simulink model "pmsm_fpga"  (R2020b)
settings: Solver=FixedStepDiscrete  StartTime=0.0  StopTime=5  FixedStep=1e-5  RelTol=1e-3
PostLoadFcn:
  | try
  | cell = struct2cell(dir(fullfile(speedgoatroot_hdlb, 'hdlsrc', 'pwm', '*.vhd')));
  | addSourceFiles = strjoin(fullfile(cell(2,:),cell(1,:)), ';');
  | hdlset_param('pwm_example_hdlc/DUT PWM and CAP', 'IPCoreAdditionalFiles', addSourceFiles);
  | end
undefined symbols (not defined in the file): J, Tmax, Ts, Tsc
libraries: fl_lib x10, nesl_utility x8, ee_lib x3, simulink x2, quadrature_cpulib x1, pwm_fpgalib x1, quadrature_fpgalib x1, eePmsmFieldOrientedControl x1, pwm_cpulib x1, eeQuadratureDecoder x1, mcbplantlib x1
settings Model: ModifiedByFormat=Speedgoat GmbH  Creator=Speedgoat GmbH  LastModifiedBy=Speedgoat GmbH
settings DataIOCC: LimitDataPoints=on  SaveFormat=Array  ReturnWorkspaceOutputs=off
settings OptimizationCC: BlockReduction=off  ConditionallyExecuteInputs=off  DefaultParameterBehavior=Inlined  LifeSpan=inf
settings DebuggingCC: AlgebraicLoopMsg=error  UnderspecifiedInitializationDetection=Classic  MergeDetectMultiDrivingBlocksExec=none  SolverPrmCheckMsg=warning  InheritedTsInSrcMsg=none  SingleTaskRateTransMsg=error  ParameterPrecisionLossMsg=none  PregeneratedLibrarySubsystemCodeDiagnostic=none  SFUnexpectedBacktrackingDiag=warning  SFNoUnconditionalDefaultTransitionDiag=warning  SFExecutionAtInitializationDiag=none  ArithmeticOperatorsInVariantConditions=warning
settings HardwareCC: ProdBitPerPointer=32  ProdBitPerSizeT=32  ProdBitPerPtrDiffT=32  ProdLargestAtomicFloat=None  ProdIntDivRoundTo=Undefined  ProdEndianess=Unspecified  ProdWordSize=32  ProdHWDeviceType=ASIC/FPGA->ASIC/FPGA  ProdEqTarget=off
settings ModelReferenceCC: PropagateSignalLabelsOutOfModel=off
settings SFSimCC: SimUseLocalCustomCode=off  CustomCodeUndefinedFunction=UseInterfaceOnly
settings RTWCC: RTWUseLocalCustomCode=off
settings CodeAppCC: StateflowObjectComments=on
settings GRTTargetCC: TargetLangStandard=C89/C90 (ANSI)
settings ConfigComp: CovMetricSettings=dw  CovSaveCumulativeToWorkspaceVar=on  CovSaveSingleToWorkspaceVar=on  CovExternalEMLEnable=off

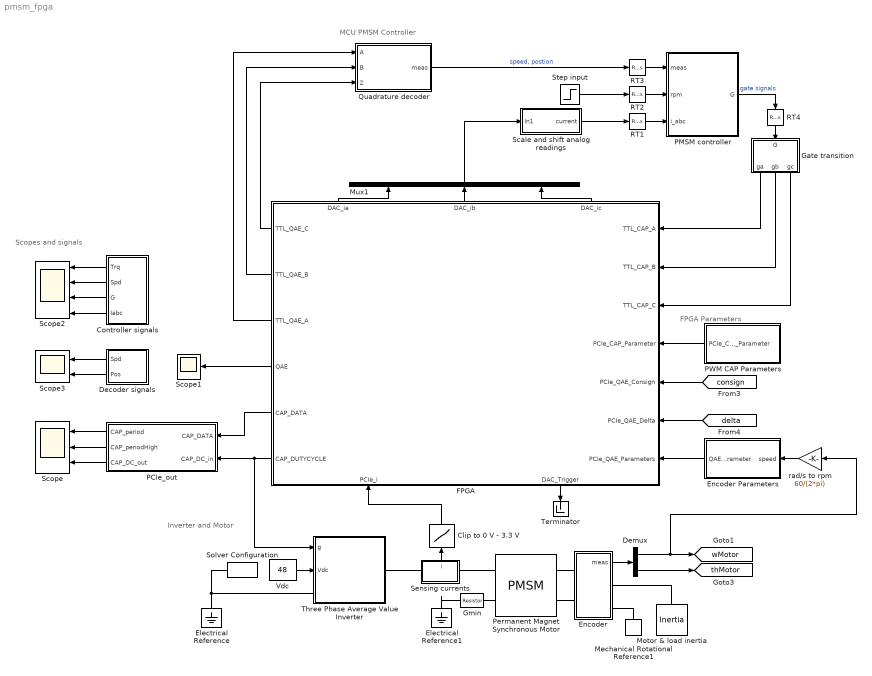
== system pmsm_fpga ==
  note: Scopes and signals
  note: Inverter and Motor
  note: FPGA Parameters
  note: MCU PMSM Controller
  Clip to 0 V - 3.3 V : Lookup_n-D  NumberOfTableDimensions=1  BreakpointsForDimension1=[0, 3.3/10*(2^15-1)]  Table=[0, 3.3/10*(2^15-1)]  ExtrapMethod=Clip  InternalRulePriority=Speed  RndMeth=Simplest  InputSameDT=on
  Controller signals : Subsystem
  Decoder signals : Subsystem
  Demux : Demux  Outputs=2
  Electrical Reference : fl_lib/Electrical/Electrical Elements/Electrical Reference
      settings: SourceProductName=Foundation Library
  Electrical Reference1 : fl_lib/Electrical/Electrical Elements/Electrical Reference
      settings: SourceProductName=Foundation Library
  Encoder : Subsystem
  Encoder Parameters : Subsystem
  FPGA : Subsystem
      settings: PortSchema="{\"entries\":[{\"content\":{\"sides\":[{\"content\":{\"connectorIds\":[\"Out5\",\"Out6\",\"Out7\",\"Out8\",\"Out9\",\"Out10\"]},\"type\":\"ConnectorPlacement.EquallySpacedRectSide\",\"uuid\":\"34ddc533-e92e-4f84-ab54-56ee31c34ed5\"},{\"content\":{\"connectorIds\":[\"In2\",\"In3\",\"In4\",\"In5\",\"In6\",\"In7\",\"In8\"],\"side\":\"RIGHT\"},\"type\":\"ConnectorPlacement.EquallySpacedRectSide\",\"uuid\":\"fc43732f-8b85-47c9-af73-b87840a05fb5\"},{\"content\":{\"connectorIds\":[\"Out2\",\"Out3\",\"Out4\"],\"side\":\"TOP\"},\"type\":\"ConnectorPlacement.EquallySpacedRectSide\",\"uuid\":\"bf663b9c-33b6-4726-afdb-56df835214b8\"},{\"content\":{\"connectorIds\":[\"In1\",\"Out1\"],\"side\":\"BOTTOM\"},\"type\":\"ConnectorPlacement.EquallySpacedRectSide\",\"uuid\":\"04fbffa8-14ef-4425-a219-a420a37a7cbf\"},{\"content\":{\"connectorIds\":[],\"side\":\"HIDDEN\"},\"type\":\"ConnectorPlacement.EquallySpacedRectSide\",\"uuid\":\"ed9b2637-afe7-435a-b994-99eac90c9c32\"}]},\"type\":\"ConnectorPlacement.EquallySpacedConnector\",\"uuid\":\"b4b9272a-3f4d-4e79-a573-4a3ad4933ba9\"}],\"packageUris\":[\"http://schema.mathworks.com/mf0/Connector/R2020b\"],\"version\":\"1.0\"}"
  Gate transition : Subsystem
  Gmin : fl_lib/Electrical/Electrical Elements/Resistor  R=1e6 Ohm  i_specify=off  i_priority=High  i=0 A  i_nominal_specify=off  i_nominal_unit=A  i_nominal_value=1  v_specify=off  v_priority=High  v=0 V  v_nominal_specify=off  v_nominal_unit=V  v_nominal_value=1
      settings: SourceProductName=Foundation Library
  Mechanical Rotational Reference1 : fl_lib/Mechanical/Rotational Elements/Mechanical Rotational Reference
      settings: SourceProductName=Foundation Library
  Motor & load inertia : fl_lib/Mechanical/Rotational Elements/Inertia  inertia=J kg*m^2  num_ports=foundation.enum.numPorts2.one  w_specify=on  w_priority=High  w=0 rpm  w_nominal_specify=off  w_nominal_unit=rad/s  w_nominal_value=1  t_specify=off  t_priority=High  t=0 N*m  t_nominal_specify=off  t_nominal_unit=N*m  t_nominal_value=1
      settings: SourceProductName=Foundation Library
  Mux1 : Mux  Inputs=3
  PCIe_out : Subsystem
  PMSM controller : Subsystem
  PWM CAP Parameters : Subsystem
  Permanent Magnet Synchronous Motor : ee_lib/Electromechanical/Permanent Magnet/PMSM  winding_type=ee.enum.statorconnection.wye  machine_param=ee.enum.pmsm.parameterization.constant  nPolePairs=N  pmflux_param=ee.enum.pmflux.fluxlinkage  pm_flux_linkage=PM Wb  torque_constant=0.18 N*m/A  back_emf_constant=0.18 V/(rad/s)  stator_param=ee.enum.statorparam.LdLqL0  Ld=Ld H  Lq=Lq H  idVec=[-200, 0, 200] A  iqVec=[-200, 0, 200] A  LdMatrix=0.0002 * ones(3, 3) H  LqMatrix=0.0002 * ones(3, 3) H  PmMatrix=0.1 * ones(3, 3) Wb  ktMatrix=0.18 * ones(3, 3) N*m/A  keMatrix=0.18 * ones(3, 3) V/(rad/s)  L0=L0 H  Ls=0.0002 H  Lm=0.00002 H  Ms=0.00002 H  Rs=Rs Ohm  zero_sequence=ee.enum.park.zerosequence.exclude  J=0 kg*m^2  lam=0 N*m/(rad/s)  axes_param=ee.enum.rotorangle.qaxis  i_d_specify=off  i_d_priority=None  i_d=0 A  i_d_nominal_specify=off  i_d_nominal_unit=A  i_d_nominal_value=1  i_q_specify=off  i_q_priority=None  i_q=0 A  i_q_nominal_specify=off  i_q_nominal_unit=A  i_q_nominal_value=1  torque_specify=off  torque_priority=None  torque=0 N*m  torque_nominal_specify=off  torque_nominal_unit=N*m  torque_nominal_value=1  angular_velocity_specify=on  angular_velocity_priority=None  angular_velocity=0 rpm  angular_velocity_nominal_specify=off  angular_velocity_nominal_unit=rpm  angular_velocity_nominal_value=1  angular_position_specify=on  angular_position_priority=High  angular_position=0 rad  angular_position_nominal_specify=off  angular_position_nominal_unit=deg  angular_position_nominal_value=1  loss_param=ee.enum.ironloss.none  losses_oc=[0, 0, 0] W  losses_sc=[0, 0, 0] W  f_losses=60 Hz  Isc_losses=95 A  Tmeas=298.15 K  alpha=3.93e-3 1/K  alpha_flux=-0.001 1/K  stator_thermal_mass=100 J/K  rotor_thermal_mass=200 J/K  Rm_percent_rotor=90  Rd_percent_rotor=30  temperatureA_specify=off  temperatureA_priority=High  temperatureA=25 degC  temperatureA_nominal_specify=off  temperatureA_nominal_unit=degC  temperatureA_nominal_value=1  temperatureB_specify=off  temperatureB_priority=High  temperatureB=25 degC  temperatureB_nominal_specify=off  temperatureB_nominal_unit=degC  temperatureB_nominal_value=1  temperatureC_specify=off  temperatureC_priority=High  temperatureC=25 degC  temperatureC_nominal_specify=off  temperatureC_nominal_unit=degC  temperatureC_nominal_value=1  temperatureR_specify=off  temperatureR_priority=High  temperatureR=25 degC  temperatureR_nominal_specify=off  temperatureR_nominal_unit=degC  temperatureR_nominal_value=1
      settings: SourceProductName=Electrical  InternalSimscapePortConfiguration="{\"Bottom\":[],\"Left\":[{\"id\":\"N\",\"label\":\"~\",\"type\":\"foundation.electrical.three_phase\"},{\"id\":\"n\",\"label\":\"n\",\"type\":\"foundation.electrical.electrical\"}],\"Right\":[{\"id\":\"R\",\"label\":\"R\",\"type\":\"foundation.mechanical.rotational.rotational\"},{\"id\":\"C\",\"label\":\"C\",\"type\":\"foundation.mechanical.rotational.rotational\"}],\"Top\":[]}"
  Quadrature decoder : Subsystem
  RT{1..4} (4 alike) : RateTransition  OutPortSampleTime=Tsc
  Scale and shift analog readings : Subsystem
  Scope : Scope  NumInputPorts=3
  Scope1 : Scope
  Scope2 : Scope  NumInputPorts=4
  Scope3 : Scope  NumInputPorts=2
  Sensing currents : Subsystem
      settings: PortSchema="{\"entries\":[{\"content\":{\"sides\":[{\"content\":{\"connectorIds\":[\"LConn1\"]},\"type\":\"ConnectorPlacement.EquallySpacedRectSide\",\"uuid\":\"5944ef88-f0e5-49d7-9ad6-739ca14af38a\"},{\"content\":{\"connectorIds\":[\"RConn1\"],\"side\":\"RIGHT\"},\"type\":\"ConnectorPlacement.EquallySpacedRectSide\",\"uuid\":\"52c09ccb-1303-4088-b38f-68b8aea00489\"},{\"content\":{\"connectorIds\":[\"Out1\"],\"side\":\"TOP\"},\"type\":\"ConnectorPlacement.EquallySpacedRectSide\",\"uuid\":\"f2e54c46-4573-400c-9f21-48a88d224d47\"},{\"content\":{\"connectorIds\":[],\"side\":\"HIDDEN\"},\"type\":\"ConnectorPlacement.EquallySpacedRectSide\",\"uuid\":\"a55d9811-d0ed-49ba-b1a1-43558df722e5\"}]},\"type\":\"ConnectorPlacement.EquallySpacedConnector\",\"uuid\":\"6a30da7c-a08b-4558-b141-c480e5507c55\"}],\"packageUris\":[\"http://schema.mathworks.com/mf0/Connector/R2020b\"],\"version\":\"1.0\"}"
      mask Display: disp('i')
  Solver Configuration : nesl_utility/Solver Configuration  PhysicalDomain=network_engine_domain  SubClassName=solver  LeftPortType=input  RightPortType=generic  Tones=[]  Harmonics=[]  SimulateNoise=off  Profile=off  UseLocalSampling=off  EnableSwitchedLinearOptims=on  FrequencyDomain=off  UseCCode=off  RelTol=0.001  AbsTol=1e-06  MinStep=1e-09  ToWorkspace=off  RevertToSquareIcSolve=off  NumHomotopyIterations=100  PhasorMode=off  PhasorModeNumHarmonics=1  DoDC=off  ResidualTolerance=1e-9  UseLocalSolver=on  LocalSolverChoice=NE_BACKWARD_EULER_ADVANCER  LocalSolverSampleTime=Ts  DoFixedCost=on  MaxNonlinIter=4  MaxModeIter=2  ComputeImpulses=off  ImpulseIterations=2  LinearAlgebra=auto  EquationFormulation=NE_TIME_EF  DelaysMemoryBudget=1024  AutomaticFiltering=on  FilteringTimeConstant=0.001  PartitionStorageMethod=AS_NEEDED  PartitionMemoryBudget=1024  PartitionMethod=FAST
      settings: SourceProductName=Utilities
  Step input : Step  Time=0.1  After=500  SampleTime=Ts
  Terminator : Terminator
  Three Phase Average Value Inverter : Subsystem
  Vdc : Constant  Value=48  SampleTime=Tsc
  rad/s to rpm : Gain  Gain=60/(2*pi)
  tag scope: thMotor=global, wMotor=global
  wires:
  PCIe_out/3(CAP_DC_out) -> Scope/3
  PCIe_out/2(CAP_periodHigh) -> Scope/2
  PCIe_out/1(CAP_period) -> Scope/1
  Encoder Parameters/1(QAE_parameter) -> FPGA/8(PCIe_QAE_Parameters)
  PWM CAP Parameters/1(PCIe_CAP_Parameter) -> FPGA/5(PCIe_CAP_Parameter)
  FPGA/10(CAP_DUTYCYCLE) -> Three Phase Average Value Inverter/1(g), PCIe_out/2(CAP_DC_in)
  FPGA/9(CAP_DATA) -> PCIe_out/1(CAP_DATA)
  Encoder/1(meas) -> Demux/1
  Vdc/1 -> Three Phase Average Value Inverter/2(Vdc)
  Demux/1 -> rad/s to rpm/1, [wMotor]
  Demux/2 -> [thMotor]
  rad/s to rpm/1 -> Encoder Parameters/1(speed)
  FPGA/8(QAE) -> Scope1/1
  RT3/1 -> PMSM controller/1(meas)
  RT2/1 -> PMSM controller/2(rpm)
  RT1/1 -> PMSM controller/3(i_abc)
  Step input/1 -> RT2/1
  FPGA/3(DAC_ib) -> Mux1/2
  FPGA/2(DAC_ia) -> Mux1/1
  FPGA/4(DAC_ic) -> Mux1/3
  FPGA/1(DAC_Trigger) -> Terminator/1
  FPGA/5(TTL_QAE_C) -> Quadrature decoder/3(Z)
  FPGA/6(TTL_QAE_B) -> Quadrature decoder/2(B)
  FPGA/7(TTL_QAE_A) -> Quadrature decoder/1(A)
  Quadrature decoder/1(meas) -> RT3/1  "speed, postion"
  Controller signals/1(Trq) -> Scope2/1
  Controller signals/2(Spd) -> Scope2/2
  Controller signals/4(Iabc) -> Scope2/4
  Controller signals/3(G) -> Scope2/3
  Decoder signals/1(Spd) -> Scope3/1
  Decoder signals/2(Pos) -> Scope3/2
  [delta] -> FPGA/7(PCIe_QAE_Delta)
  [consign] -> FPGA/6(PCIe_QAE_Consign)
  PMSM controller/1(G) -> RT4/1  "gate signals"
  Gate transition/1(ga) -> FPGA/2(TTL_CAP_A)
  Gate transition/2(gb) -> FPGA/3(TTL_CAP_B)
  Gate transition/3(gc) -> FPGA/4(TTL_CAP_C)
  Sensing currents/1(i) -> Clip to 0 V - 3.3 V/1
  Clip to 0 V - 3.3 V/1 -> FPGA/1(PCIe_i)
  Mux1/1 -> Scale and shift analog readings/1(In1)
  Scale and shift analog readings/1(current) -> RT1/1
  RT4/1 -> Gate transition/1(G)
  connections:
  Solver Configuration/RConn1 -- Electrical Reference/LConn1 -- Three Phase Average Value Inverter/LConn1
  Electrical Reference1/LConn1 -- Gmin/LConn1
  Encoder/RConn1 -- Motor & load inertia/LConn1
  Permanent Magnet Synchronous Motor/RConn1 -- Encoder/LConn1
  Three Phase Average Value Inverter/RConn1 -- Sensing currents/LConn1
  Permanent Magnet Synchronous Motor/RConn2 -- Encoder/LConn2
  Mechanical Rotational Reference1/LConn1 -- Encoder/RConn2
  Permanent Magnet Synchronous Motor/LConn1 -- Sensing currents/RConn1
  Gmin/RConn1 -- Permanent Magnet Synchronous Motor/LConn2

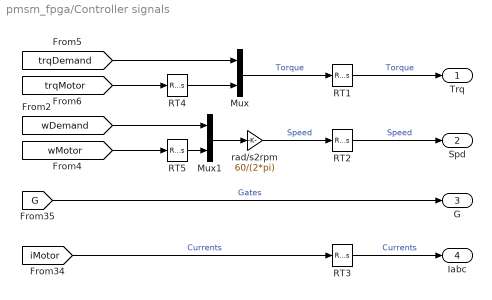
== system pmsm_fpga/Controller signals ==
  Mux : Mux  Inputs=2
  Mux1 : Mux  Inputs=2
  RT1 : RateTransition  OutPortSampleTime=Ts
  RT2 : RateTransition  OutPortSampleTime=Ts
  RT3 : RateTransition  OutPortSampleTime=Ts
  RT4 : RateTransition  OutPortSampleTime=Tsc
  RT5 : RateTransition  OutPortSampleTime=Tsc
  rad/s2rpm : Gain  Gain=60/(2*pi)
  Trq : Outport  VectorParamsAs1DForOutWhenUnconnected=off
  Spd : Outport  Port=2  VectorParamsAs1DForOutWhenUnconnected=off
  G : Outport  Port=3  VectorParamsAs1DForOutWhenUnconnected=off
  Iabc : Outport  Port=4  VectorParamsAs1DForOutWhenUnconnected=off
  wires:
  [trqDemand] -> Mux/1
  [G] -> G/1  "Gates"
  Mux1/1 -> rad/s2rpm/1
  Mux/1 -> RT1/1  "Torque"
  [iMotor] -> RT3/1  "Currents"
  [wDemand] -> Mux1/1
  rad/s2rpm/1 -> RT2/1  "Speed"
  [trqMotor] -> RT4/1
  [wMotor] -> RT5/1
  RT1/1 -> Trq/1  "Torque"
  RT2/1 -> Spd/1  "Speed"
  RT3/1 -> Iabc/1  "Currents"
  RT4/1 -> Mux/2
  RT5/1 -> Mux1/2

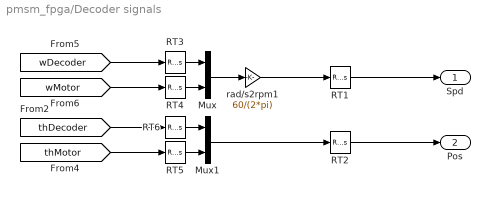
== system pmsm_fpga/Decoder signals ==
  Mux : Mux  Inputs=2
  Mux1 : Mux  Inputs=2
  RT1 : RateTransition  OutPortSampleTime=Ts
  RT2 : RateTransition  OutPortSampleTime=Ts
  RT{3..6} (4 alike) : RateTransition  OutPortSampleTime=Tsc
  rad/s2rpm1 : Gain  Gain=60/(2*pi)
  Spd : Outport  VectorParamsAs1DForOutWhenUnconnected=off
  Pos : Outport  Port=2  VectorParamsAs1DForOutWhenUnconnected=off
  wires:
  [wDecoder] -> RT3/1
  Mux/1 -> rad/s2rpm1/1
  [thDecoder] -> RT6/1
  Mux1/1 -> RT2/1
  [wMotor] -> RT4/1
  [thMotor] -> RT5/1
  RT1/1 -> Spd/1
  RT2/1 -> Pos/1
  RT4/1 -> Mux/2
  RT5/1 -> Mux1/2
  rad/s2rpm1/1 -> RT1/1
  RT3/1 -> Mux/1
  RT6/1 -> Mux1/1

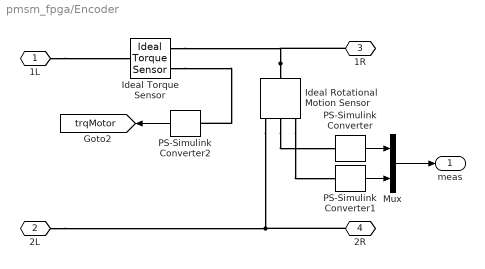
== system pmsm_fpga/Encoder ==
  Ideal Rotational Motion Sensor : fl_lib/Mechanical/Mechanical Sensors/Ideal Rotational Motion Sensor  wrap_angle=simscape.enum.onoff.off  offset=0 deg
      settings: SourceProductName=Foundation Library
  Ideal Torque Sensor : fl_lib/Mechanical/Mechanical Sensors/Ideal Torque Sensor
      settings: SourceProductName=Foundation Library
  Mux : Mux  Inputs=2
  PS-Simulink Converter : nesl_utility/PS-Simulink Converter  PhysicalDomain=network_engine_domain  SubClassName=ps_output  LeftPortType=input  RightPortType=output  PseudoPeriodic=off  Frequencies=[]  Unit=rad/s  AffineConversion=off
      settings: SourceProductName=Utilities
  PS-Simulink Converter1 : nesl_utility/PS-Simulink Converter  PhysicalDomain=network_engine_domain  SubClassName=ps_output  LeftPortType=input  RightPortType=output  PseudoPeriodic=off  Frequencies=[]  Unit=rad  AffineConversion=off
      settings: SourceProductName=Utilities
  PS-Simulink Converter2 : nesl_utility/PS-Simulink Converter  PhysicalDomain=network_engine_domain  SubClassName=ps_output  LeftPortType=input  RightPortType=output  PseudoPeriodic=off  Frequencies=[]  Unit=N*m  AffineConversion=off
      settings: SourceProductName=Utilities
  1L : PMIOPort  Side=Left
  2L : PMIOPort  Port=2  Side=Left
  1R : PMIOPort  Port=3  Side=Right
  2R : PMIOPort  Port=4  Side=Right
  meas : Outport  VectorParamsAs1DForOutWhenUnconnected=off
  tag scope: trqMotor=global
  wires:
  PS-Simulink Converter2/1 -> [trqMotor]
  Mux/1 -> meas/1
  PS-Simulink Converter1/1 -> Mux/2
  PS-Simulink Converter/1 -> Mux/1
  connections:
  Ideal Torque Sensor/RConn2 -- PS-Simulink Converter2/LConn1
  1L/RConn1 -- Ideal Torque Sensor/LConn1
  2R/RConn1 -- 2L/RConn1 -- Ideal Rotational Motion Sensor/RConn1
  Ideal Rotational Motion Sensor/LConn1 -- 1R/RConn1 -- Ideal Torque Sensor/RConn1
  Ideal Rotational Motion Sensor/RConn2 -- PS-Simulink Converter/LConn1
  Ideal Rotational Motion Sensor/RConn3 -- PS-Simulink Converter1/LConn1

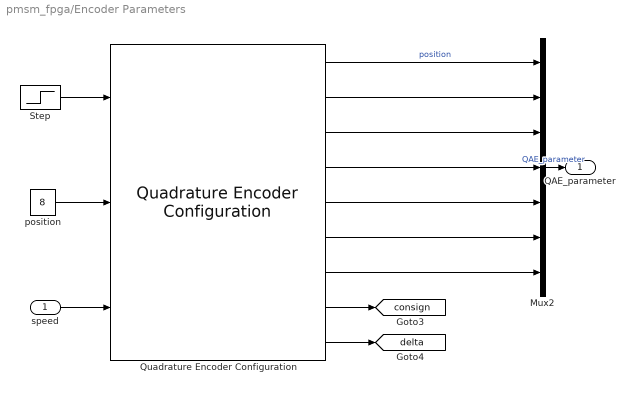
== system pmsm_fpga/Encoder Parameters ==
  speed : Inport
  Mux2 : Mux  Inputs=7
  Quadrature Encoder Configuration : quadrature_cpulib/Quadrature Encoder Configuration  fpgaFreq=100e6  n_channels=1  numSeg=[32]  phaseAngle=90  initPos=[0]  freeWheel=on
      settings: SourceProductName=Simulink Real-Time: Speedgoat HDL Blockset
  Step : Step  Time=0.002
  position : Constant  Value=8  SampleTime=-1
  QAE_parameter : Outport
  tag scope: consign=global, delta=global
  wires:
  speed/1 -> Quadrature Encoder Configuration/3
  Quadrature Encoder Configuration/8 -> [consign]
  Step/1 -> Quadrature Encoder Configuration/1
  Quadrature Encoder Configuration/7 -> Mux2/7
  Quadrature Encoder Configuration/4 -> Mux2/4
  Quadrature Encoder Configuration/2 -> Mux2/2
  position/1 -> Quadrature Encoder Configuration/2
  Mux2/1 -> QAE_parameter/1  "QAE_parameter"
  Quadrature Encoder Configuration/6 -> Mux2/6
  Quadrature Encoder Configuration/5 -> Mux2/5
  Quadrature Encoder Configuration/1 -> Mux2/1  "position"
  Quadrature Encoder Configuration/9 -> [delta]
  Quadrature Encoder Configuration/3 -> Mux2/3

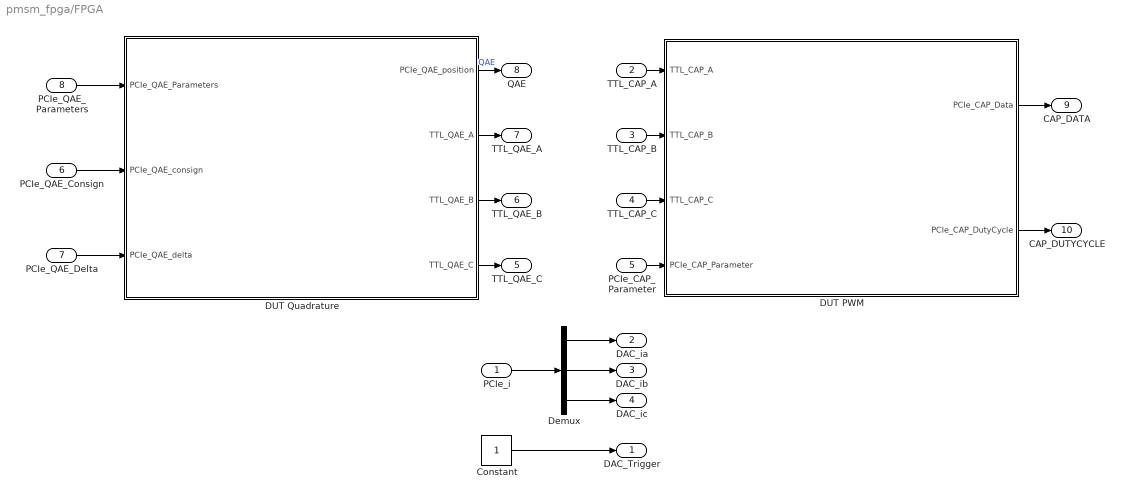
== system pmsm_fpga/FPGA ==
  PCIe_i : Inport  OutDataTypeStr=int16
  TTL_CAP_A : Inport  Port=2
  TTL_CAP_B : Inport  Port=3
  TTL_CAP_C : Inport  Port=4
  PCIe_CAP_Parameter : Inport  Port=5
  PCIe_QAE_Consign : Inport  Port=6
  PCIe_QAE_Delta : Inport  Port=7
  PCIe_QAE_Parameters : Inport  Port=8
  Constant : Constant  OutDataTypeStr=boolean  SampleTime=-1
  DUT PWM : Subsystem
  DUT Quadrature : Subsystem
  Demux : Demux  Outputs=3
  DAC_Trigger : Outport
  DAC_ia : Outport  Port=2
  DAC_ib : Outport  Port=3
  DAC_ic : Outport  Port=4
  TTL_QAE_C : Outport  Port=5
  TTL_QAE_B : Outport  Port=6
  TTL_QAE_A : Outport  Port=7
  QAE : Outport  Port=8
  CAP_DATA : Outport  Port=9
  CAP_DUTYCYCLE : Outport  Port=10
  wires:
  PCIe_QAE_Parameters/1 -> DUT Quadrature/1(PCIe_QAE_Parameters)
  TTL_CAP_B/1 -> DUT PWM/2(TTL_CAP_B)
  PCIe_QAE_Consign/1 -> DUT Quadrature/2(PCIe_QAE_consign)
  PCIe_CAP_Parameter/1 -> DUT PWM/4(PCIe_CAP_Parameter)
  PCIe_QAE_Delta/1 -> DUT Quadrature/3(PCIe_QAE_delta)
  DUT Quadrature/3(TTL_QAE_B) -> TTL_QAE_B/1
  DUT PWM/1(PCIe_CAP_Data) -> CAP_DATA/1
  TTL_CAP_C/1 -> DUT PWM/3(TTL_CAP_C)
  DUT Quadrature/4(TTL_QAE_C) -> TTL_QAE_C/1
  DUT Quadrature/1(PCIe_QAE_position) -> QAE/1  "QAE"
  DUT Quadrature/2(TTL_QAE_A) -> TTL_QAE_A/1
  DUT PWM/2(PCIe_CAP_DutyCycle) -> CAP_DUTYCYCLE/1
  TTL_CAP_A/1 -> DUT PWM/1(TTL_CAP_A)
  PCIe_i/1 -> Demux/1
  Demux/1 -> DAC_ia/1
  Demux/2 -> DAC_ib/1
  Demux/3 -> DAC_ic/1
  Constant/1 -> DAC_Trigger/1

== system pmsm_fpga/Gate transition ==
  G : Inport
  Demux1 : Demux  Outputs=6
  Terminator1 : Terminator
  Terminator2 : Terminator
  Terminator3 : Terminator
  ga : Outport
  gb : Outport  Port=2
  gc : Outport  Port=3
  wires:
  Demux1/2 -> Terminator1/1
  Demux1/6 -> Terminator3/1
  G/1 -> Demux1/1
  Demux1/4 -> Terminator2/1
  Demux1/1 -> ga/1
  Demux1/3 -> gb/1
  Demux1/5 -> gc/1

== system pmsm_fpga/PCIe_out ==
  CAP_DATA : Inport
  CAP_DC_in : Inport  Port=2
  Bus Creator : BusCreator  Inputs=6
  Bus Selector : BusSelector  OutputSignals=PCIe_CAP_Period,PCIe_CAP_periodHigh
  Demux : Demux  Outputs=6
  CAP_period : Outport
  CAP_periodHigh : Outport  Port=2
  CAP_DC_out : Outport  Port=3
  wires:
  CAP_DC_in/1 -> CAP_DC_out/1  "CAP_DutyCycle"
  Bus Selector/2 -> CAP_periodHigh/1  "<PCIe_CAP_periodHigh>"
  Bus Selector/1 -> CAP_period/1  "<PCIe_CAP_Period>"
  Demux/6 -> Bus Creator/6  "PCIe_CAP_Data_Valid"
  Demux/3 -> Bus Creator/3  "PCIe_CAP_periodLow"
  Demux/2 -> Bus Creator/2  "PCIe_CAP_periodHigh"
  Demux/4 -> Bus Creator/4  "PCIe_CAP_TOn"
  Bus Creator/1 -> Bus Selector/1
  Demux/1 -> Bus Creator/1  "PCIe_CAP_Period"
  Demux/5 -> Bus Creator/5  "PCIe_CAP_TOff"
  CAP_DATA/1 -> Demux/1

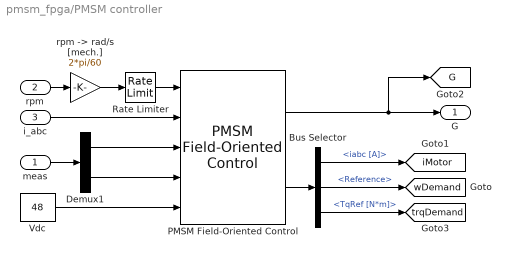
== system pmsm_fpga/PMSM controller ==
  meas : Inport
  rpm : Inport  Port=2
  i_abc : Inport  Port=3
  Bus Selector : BusSelector  OutputSignals=iabc [A],Reference,TqRef [N*m]
  Demux1 : Demux  Outputs=2
  PMSM Field-Oriented Control : eePmsmFieldOrientedControl/PMSM Field-Oriented Control  winding_type=Wye-wound  CtrlMode=Velocity control  Vnom=48  Pmax=Pmax  Tmax=Tmax*1.5  p=N  Vdc_on=10  Ts=Ts  Tsc=Tsc  CtrlType=PI control  Kp_w=60  Ki_w=300*2  Kv_w=1  Kaw_w=1000  RefType=Zero d-axis control  rpmVec=[0, 3000]  TqVec=[-100, 0, 100]  VdcVec=[300, 350]  PWMMode=SPWM: sinusoidal PWM  ModFactor=1  idMatrix=zeros(2,3,2)  iqMatrix=zeros(2,3,2)  psim=PM  Ld=0.00024  Lq=0.00029  Rs=0.01  AxisAlignment=Q-axis  Kp_id=0.1  Ki_id=10  Kaw_id=1000  Kp_iq=0.1  Ki_iq=10  Kaw_iq=1000  AxisPrio=Q-axis  ActZC=off  ActFF=on  ParamTypeFF=Constant parameters  LdFF=Ld  LqFF=Lq  psimFF=PM  idVect=[-200, 0, 200]  iqVect=[-200, 0, 200]  LdMatrix=0.0002 * ones(3, 3)  LqMatrix=0.0002 * ones(3, 3)  psimMatrix=0.04 * ones(3, 3)  CPWMMode=SPWM: sinusoidal PWM  fsw=fsw
      settings: SourceProductBaseCode=PS
  Rate Limiter : RateLimiter  RisingSlewLimit=Tmax/J  FallingSlewLimit=-Tmax/J  SampleTimeMode=inherited
  Vdc : Constant  Value=48  SampleTime=Tsc
  "rpm -> rad/s [mech.]" : Gain  Gain=2*pi/60
  G : Outport  VectorParamsAs1DForOutWhenUnconnected=off
  tag scope: G=global, iMotor=global, trqDemand=global, wDemand=global
  wires:
  PMSM Field-Oriented Control/1 -> G/1, [G]
  Vdc/1 -> PMSM Field-Oriented Control/5
  PMSM Field-Oriented Control/2 -> Bus Selector/1
  i_abc/1 -> PMSM Field-Oriented Control/2
  meas/1 -> Demux1/1
  Demux1/1 -> PMSM Field-Oriented Control/3
  Demux1/2 -> PMSM Field-Oriented Control/4
  Bus Selector/1 -> [iMotor]  "<iabc [A]>"
  Bus Selector/2 -> [wDemand]  "<Reference>"
  Bus Selector/3 -> [trqDemand]  "<TqRef [N*m]>"
  rpm/1 -> "rpm -> rad/s [mech.]"/1
  Rate Limiter/1 -> PMSM Field-Oriented Control/1
  "rpm -> rad/s [mech.]"/1 -> Rate Limiter/1

== system pmsm_fpga/PWM CAP Parameters ==
  Data Type Conversion4 : DataTypeConversion  OutDataTypeStr=uint32
  Data Type Conversion5 : DataTypeConversion  OutDataTypeStr=uint32
  Data Type Conversion6 : DataTypeConversion  OutDataTypeStr=uint32
  Mux1 : Mux  Inputs=3
  PWM Capture Configuration : pwm_cpulib/PWM Capture Configuration  FPGA_freq=100e6  n_channels=1  captureMode=High transitions triggered  captureTimeout=0  PWM_pattern_en=off
      settings: SourceProductName=Simulink Real-Time: Speedgoat HDL Blockset
  PCIe_CAP_Parameter : Outport
  wires:
  PWM Capture Configuration/2 -> Data Type Conversion5/1
  Data Type Conversion6/1 -> Mux1/3
  Data Type Conversion5/1 -> Mux1/2
  Data Type Conversion4/1 -> Mux1/1
  PWM Capture Configuration/3 -> Data Type Conversion6/1
  Mux1/1 -> PCIe_CAP_Parameter/1
  PWM Capture Configuration/1 -> Data Type Conversion4/1

== system pmsm_fpga/Quadrature decoder ==
  A : Inport
  B : Inport  Port=2
  Z : Inport  Port=3
  Mux : Mux  Inputs=2
  Quadrature Shaft Decoder : eeQuadratureDecoder/Quadrature Shaft Decoder  NPulse=16  Ts=-1
      settings: SourceProductBaseCode=PS
  meas : Outport
  tag scope: thDecoder=global, wDecoder=global
  wires:
  Z/1 -> Quadrature Shaft Decoder/3
  B/1 -> Quadrature Shaft Decoder/2
  Quadrature Shaft Decoder/1 -> Mux/1, [wDecoder]
  Mux/1 -> meas/1
  Quadrature Shaft Decoder/2 -> Mux/2, [thDecoder]
  A/1 -> Quadrature Shaft Decoder/1

== system pmsm_fpga/Scale and shift analog readings ==
  In1 : Inport
  Data Type Conversion : DataTypeConversion  OutDataTypeStr=double
  Scale to max range : Gain  Gain=20/3.3
  Shift to allow negative current : Bias  Bias=-2^15
  current : Outport
  wires:
  Scale to max range/1 -> Shift to allow negative current/1
  Data Type Conversion/1 -> Scale to max range/1
  In1/1 -> Data Type Conversion/1
  Shift to allow negative current/1 -> current/1  "current"

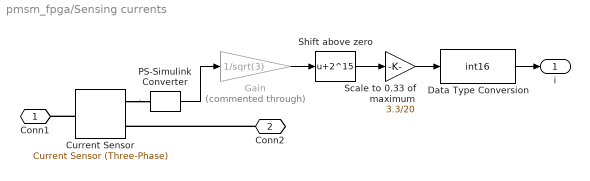
== system pmsm_fpga/Sensing currents ==
  Current Sensor : ee_lib/Sensors & Transducers/Current Sensor (Three-Phase)
      settings: SourceProductName=Electrical
  Data Type Conversion : DataTypeConversion  OutDataTypeStr=int16
  Gain : Gain  Commented=through  Gain=1/sqrt(3)
  PS-Simulink Converter : nesl_utility/PS-Simulink Converter  PhysicalDomain=network_engine_domain  SubClassName=ps_output  LeftPortType=input  RightPortType=output  PseudoPeriodic=off  Frequencies=[]  Unit=A  AffineConversion=off
      settings: SourceProductName=Utilities
  Scale to 0.33 of maximum : Gain  Gain=3.3/20
  Shift above zero : Bias  Bias=2^15
  Conn1 : PMIOPort  Side=Left
  Conn2 : PMIOPort  Port=2  Side=Right
  i : Outport
  wires:
  PS-Simulink Converter/1 -> Gain/1
  Scale to 0.33 of maximum/1 -> Data Type Conversion/1
  Data Type Conversion/1 -> i/1
  Gain/1 -> Shift above zero/1
  Shift above zero/1 -> Scale to 0.33 of maximum/1
  connections:
  Current Sensor/RConn1 -- PS-Simulink Converter/LConn1
  Conn2/RConn1 -- Current Sensor/RConn2
  Current Sensor/LConn1 -- Conn1/RConn1

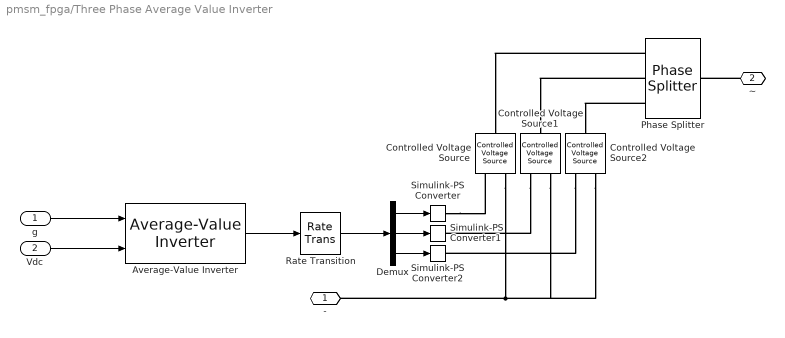
== system pmsm_fpga/Three Phase Average Value Inverter ==
  g : Inport
  Vdc : Inport  Port=2
  Average-Value Inverter : mcbplantlib/Average-Value Inverter
  Controlled Voltage Source : fl_lib/Electrical/Electrical Sources/Controlled Voltage Source
  Controlled Voltage Source1 : fl_lib/Electrical/Electrical Sources/Controlled Voltage Source
  Controlled Voltage Source2 : fl_lib/Electrical/Electrical Sources/Controlled Voltage Source
  Demux : Demux  Outputs=3
  Phase Splitter : ee_lib/Connectors & References/Phase Splitter
      settings: SourceProductBaseCode=PS
  Rate Transition : RateTransition
  Simulink-PS Converter : nesl_utility/Simulink-PS Converter  PhysicalDomain=network_engine_domain  SubClassName=ps_input  LeftPortType=input  RightPortType=output  PseudoPeriodic=off  Frequencies=[]  NoiseDistribution=none  NoiseParameters=[]  Unit=1  AffineConversion=off  FilteringAndDerivatives=provide  SimscapeFilterOrder=1  InputFilterTimeConstant=0.001  UdotUserProvided=0
  Simulink-PS Converter1 : nesl_utility/Simulink-PS Converter  PhysicalDomain=network_engine_domain  SubClassName=ps_input  LeftPortType=input  RightPortType=output  PseudoPeriodic=off  Frequencies=[]  NoiseDistribution=none  NoiseParameters=[]  Unit=1  AffineConversion=off  FilteringAndDerivatives=provide  SimscapeFilterOrder=1  InputFilterTimeConstant=0.001  UdotUserProvided=0
  Simulink-PS Converter2 : nesl_utility/Simulink-PS Converter  PhysicalDomain=network_engine_domain  SubClassName=ps_input  LeftPortType=input  RightPortType=output  PseudoPeriodic=off  Frequencies=[]  NoiseDistribution=none  NoiseParameters=[]  Unit=1  AffineConversion=off  FilteringAndDerivatives=provide  SimscapeFilterOrder=1  InputFilterTimeConstant=0.001  UdotUserProvided=0
  - : PMIOPort  Tag=PMCPort  Side=Left
  ~ : PMIOPort  Tag=PMCPort  Port=2  Side=Right
  wires:
  Demux/3 -> Simulink-PS Converter2/1
  Vdc/1 -> Average-Value Inverter/2
  Demux/2 -> Simulink-PS Converter1/1
  Demux/1 -> Simulink-PS Converter/1
  g/1 -> Average-Value Inverter/1
  Rate Transition/1 -> Demux/1
  Average-Value Inverter/1 -> Rate Transition/1
  connections:
  ~/RConn1 -- Phase Splitter/LConn1
  Controlled Voltage Source/RConn2 -- -/RConn1 -- Controlled Voltage Source1/RConn2 -- Controlled Voltage Source2/RConn2
  Simulink-PS Converter/RConn1 -- Controlled Voltage Source/RConn1
  Controlled Voltage Source2/RConn1 -- Simulink-PS Converter2/RConn1
  Phase Splitter/RConn3 -- Controlled Voltage Source2/LConn1
  Phase Splitter/RConn1 -- Controlled Voltage Source/LConn1
  Phase Splitter/RConn2 -- Controlled Voltage Source1/LConn1
  Controlled Voltage Source1/RConn1 -- Simulink-PS Converter1/RConn1

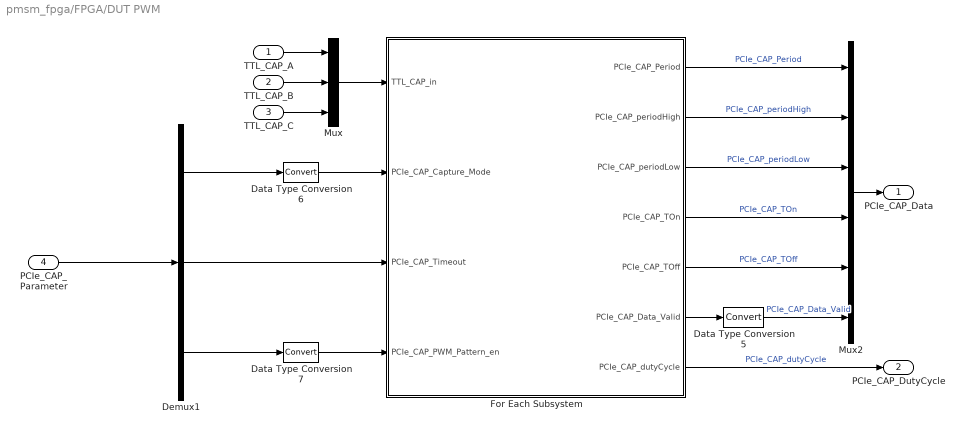
== system pmsm_fpga/FPGA/DUT PWM ==
  TTL_CAP_A : Inport
  TTL_CAP_B : Inport  Port=2
  TTL_CAP_C : Inport  Port=3
  PCIe_CAP_Parameter : Inport  Port=4
  Data Type Conversion5 : DataTypeConversion
  Data Type Conversion6 : DataTypeConversion
  Data Type Conversion7 : DataTypeConversion
  Demux1 : Demux  Outputs=3
  For Each Subsystem : Subsystem  TreatAsAtomicUnit=on
  Mux : Mux  Inputs=3
  Mux2 : Mux  Inputs=6
  PCIe_CAP_Data : Outport  VectorParamsAs1DForOutWhenUnconnected=off
  PCIe_CAP_DutyCycle : Outport  Port=2  VectorParamsAs1DForOutWhenUnconnected=off
  wires:
  Demux1/1 -> Data Type Conversion6/1
  TTL_CAP_A/1 -> Mux/1
  For Each Subsystem/7(PCIe_CAP_dutyCycle) -> PCIe_CAP_DutyCycle/1  "PCIe_CAP_dutyCycle"
  Demux1/2 -> For Each Subsystem/3(PCIe_CAP_Timeout)
  Demux1/3 -> Data Type Conversion7/1
  For Each Subsystem/6(PCIe_CAP_Data_Valid) -> Data Type Conversion5/1
  For Each Subsystem/5(PCIe_CAP_TOff) -> Mux2/5  "PCIe_CAP_TOff"
  For Each Subsystem/4(PCIe_CAP_TOn) -> Mux2/4  "PCIe_CAP_TOn"
  For Each Subsystem/3(PCIe_CAP_periodLow) -> Mux2/3  "PCIe_CAP_periodLow"
  For Each Subsystem/1(PCIe_CAP_Period) -> Mux2/1  "PCIe_CAP_Period"
  For Each Subsystem/2(PCIe_CAP_periodHigh) -> Mux2/2  "PCIe_CAP_periodHigh"
  Mux/1 -> For Each Subsystem/1(TTL_CAP_in)
  TTL_CAP_B/1 -> Mux/2
  Mux2/1 -> PCIe_CAP_Data/1
  Data Type Conversion5/1 -> Mux2/6  "PCIe_CAP_Data_Valid"
  PCIe_CAP_Parameter/1 -> Demux1/1
  Data Type Conversion6/1 -> For Each Subsystem/2(PCIe_CAP_Capture_Mode)
  Data Type Conversion7/1 -> For Each Subsystem/4(PCIe_CAP_PWM_Pattern_en)
  TTL_CAP_C/1 -> Mux/3

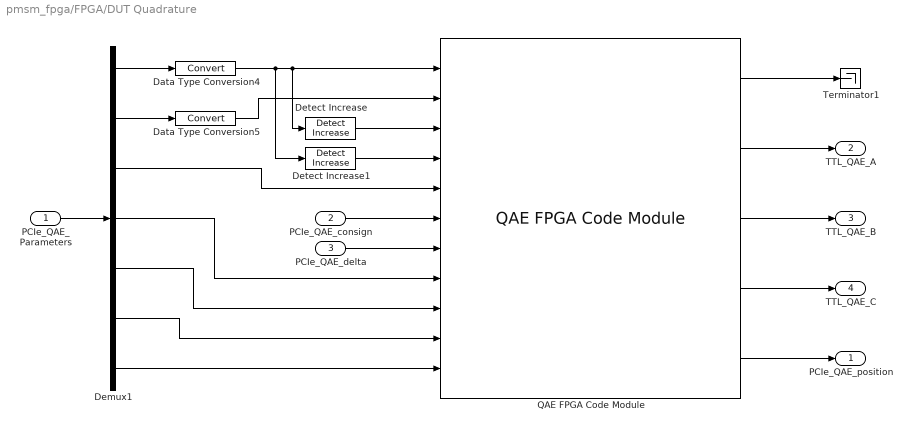
== system pmsm_fpga/FPGA/DUT Quadrature ==
  PCIe_QAE_Parameters : Inport
  PCIe_QAE_consign : Inport  Port=2  OutDataTypeStr=uint32  PortDimensions=1
  PCIe_QAE_delta : Inport  Port=3  PortDimensions=1
  Data Type Conversion4 : DataTypeConversion
  Data Type Conversion5 : DataTypeConversion
  Demux1 : Demux  Outputs=7
  Detect Increase : simulink/Logic and Bit Operations/Detect Increase  vinit=0.0  OutDataTypeStr=boolean
  Detect Increase1 : simulink/Logic and Bit Operations/Detect Increase  vinit=0.0  OutDataTypeStr=boolean
  QAE FPGA Code Module : quadrature_fpgalib/QAE FPGA Code Module  SystemSampleTime=-1  VariantActivationTime=update diagram  Latency=0  AutoFrameSizeCalculation=off
      settings: SourceProductName=Simulink Real-Time: Speedgoat Functionality Package
  Terminator1 : Terminator
  PCIe_QAE_position : Outport  VectorParamsAs1DForOutWhenUnconnected=off
  TTL_QAE_A : Outport  Port=2  VectorParamsAs1DForOutWhenUnconnected=off
  TTL_QAE_B : Outport  Port=3  VectorParamsAs1DForOutWhenUnconnected=off
  TTL_QAE_C : Outport  Port=4  VectorParamsAs1DForOutWhenUnconnected=off
  wires:
  QAE FPGA Code Module/5 -> PCIe_QAE_position/1
  Detect Increase1/1 -> QAE FPGA Code Module/4
  Detect Increase/1 -> QAE FPGA Code Module/3
  QAE FPGA Code Module/4 -> TTL_QAE_C/1
  QAE FPGA Code Module/2 -> TTL_QAE_A/1
  QAE FPGA Code Module/3 -> TTL_QAE_B/1
  PCIe_QAE_delta/1 -> QAE FPGA Code Module/7
  QAE FPGA Code Module/1 -> Terminator1/1
  PCIe_QAE_consign/1 -> QAE FPGA Code Module/6
  Demux1/1 -> Data Type Conversion4/1
  Demux1/2 -> Data Type Conversion5/1
  Demux1/3 -> QAE FPGA Code Module/5
  Demux1/4 -> QAE FPGA Code Module/8
  Demux1/5 -> QAE FPGA Code Module/9
  PCIe_QAE_Parameters/1 -> Demux1/1
  Data Type Conversion4/1 -> Detect Increase1/1, QAE FPGA Code Module/1, Detect Increase/1
  Data Type Conversion5/1 -> QAE FPGA Code Module/2
  Demux1/6 -> QAE FPGA Code Module/10
  Demux1/7 -> QAE FPGA Code Module/11

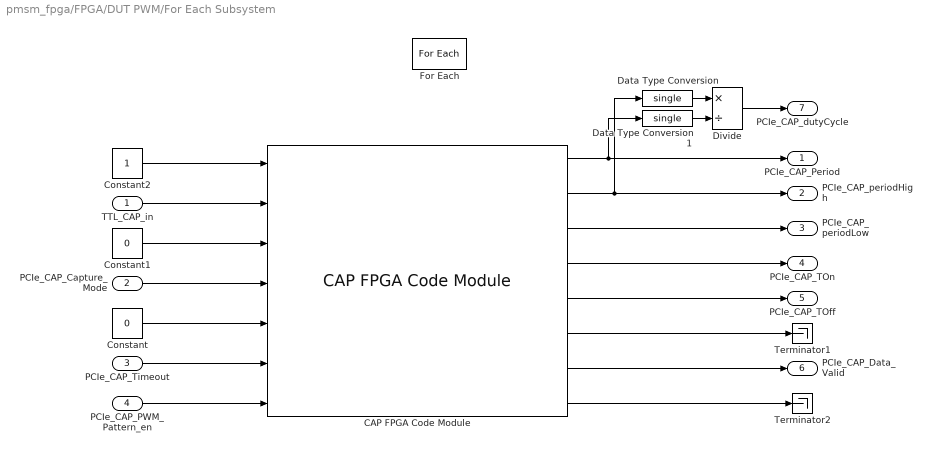
== system pmsm_fpga/FPGA/DUT PWM/For Each Subsystem ==
  TTL_CAP_in : Inport  Partition=on  PartitionDimension=1  PartitionWidth=1  PartitionOffset=0
  PCIe_CAP_Capture_Mode : Inport  Port=2
  PCIe_CAP_Timeout : Inport  Port=3
  PCIe_CAP_PWM_Pattern_en : Inport  Port=4
  CAP FPGA Code Module : pwm_fpgalib/CAP FPGA Code Module  SystemSampleTime=-1  VariantActivationTime=update diagram  Latency=0  AutoFrameSizeCalculation=off
      settings: SourceProductName=Simulink Real-Time: Speedgoat Functionality Package
  Constant : Constant  Value=0  OutDataTypeStr=Inherit: Inherit via back propagation  SampleTime=-1
  Constant1 : Constant  Value=0  OutDataTypeStr=Inherit: Inherit via back propagation  SampleTime=-1
  Constant2 : Constant  OutDataTypeStr=Inherit: Inherit via back propagation  SampleTime=-1
  Data Type Conversion : DataTypeConversion  OutMin=0  OutDataTypeStr=single
  Data Type Conversion1 : DataTypeConversion  OutMin=0  OutDataTypeStr=single  LockScale=on
  Divide : Product  Inputs=*/  RndMeth=Zero  SaturateOnIntegerOverflow=on
  For Each : ForEach  DisableCoverage=on
  Terminator1 : Terminator
  Terminator2 : Terminator
  PCIe_CAP_Period : Outport  ConcatenationDimension=2  VectorParamsAs1DForOutWhenUnconnected=off
  PCIe_CAP_periodHigh : Outport  Port=2  ConcatenationDimension=2  VectorParamsAs1DForOutWhenUnconnected=off
  PCIe_CAP_periodLow : Outport  Port=3  ConcatenationDimension=2  VectorParamsAs1DForOutWhenUnconnected=off
  PCIe_CAP_TOn : Outport  Port=4  ConcatenationDimension=2  VectorParamsAs1DForOutWhenUnconnected=off
  PCIe_CAP_TOff : Outport  Port=5  ConcatenationDimension=2  VectorParamsAs1DForOutWhenUnconnected=off
  PCIe_CAP_Data_Valid : Outport  Port=6  ConcatenationDimension=2  VectorParamsAs1DForOutWhenUnconnected=off
  PCIe_CAP_dutyCycle : Outport  Port=7  ConcatenationDimension=2  VectorParamsAs1DForOutWhenUnconnected=off
  wires:
  Data Type Conversion/1 -> Divide/1
  Divide/1 -> PCIe_CAP_dutyCycle/1
  Constant1/1 -> CAP FPGA Code Module/3
  PCIe_CAP_Capture_Mode/1 -> CAP FPGA Code Module/4
  Constant/1 -> CAP FPGA Code Module/5
  TTL_CAP_in/1 -> CAP FPGA Code Module/2
  PCIe_CAP_Timeout/1 -> CAP FPGA Code Module/6
  PCIe_CAP_PWM_Pattern_en/1 -> CAP FPGA Code Module/7
  Constant2/1 -> CAP FPGA Code Module/1
  CAP FPGA Code Module/3 -> PCIe_CAP_periodLow/1
  CAP FPGA Code Module/8 -> Terminator2/1
  CAP FPGA Code Module/5 -> PCIe_CAP_TOff/1
  CAP FPGA Code Module/6 -> Terminator1/1
  CAP FPGA Code Module/2 -> PCIe_CAP_periodHigh/1, Data Type Conversion/1
  CAP FPGA Code Module/7 -> PCIe_CAP_Data_Valid/1
  CAP FPGA Code Module/1 -> PCIe_CAP_Period/1, Data Type Conversion1/1
  CAP FPGA Code Module/4 -> PCIe_CAP_TOn/1
  Data Type Conversion1/1 -> Divide/2
